simulink model "controlPC2"  (R2015b)
settings: Solver=ode45  StartTime=0.0  StopTime=100  RelTol=1e-3
values from neighbouring files (symbols this model uses):
  Kf = 20    [parametros.m]    (also in ploteo.m)
  Kpi = 0.014    [parametros.m]    (also in ploteo.m)
  T = 0.04    [parametros.m]    (also in ploteo.m)
  Ti = 0.25    [parametros.m]    (also in ploteo.m)
settings Model: Creator=Sony  LastModifiedBy=n421
settings DataIOCC: SaveFormat=Array
settings OptimizationCC: ExpressionDepthLimit=2147483647
settings DebuggingCC: UnderspecifiedInitializationDetection=Classic  MergeDetectMultiDrivingBlocksExec=none  SolverPrmCheckMsg=warning  StateNameClashWarn=warning
settings HardwareCC: ProdBitPerPointer=32  ProdLargestAtomicFloat=None  ProdIntDivRoundTo=Undefined  ProdEndianess=Unspecified  ProdWordSize=32  ProdHWDeviceType=32-bit Generic
settings GRTTargetCC: GeneratePreprocessorConditionals=Disable all
settings ConfigComp: CovModelRefEnable=Off

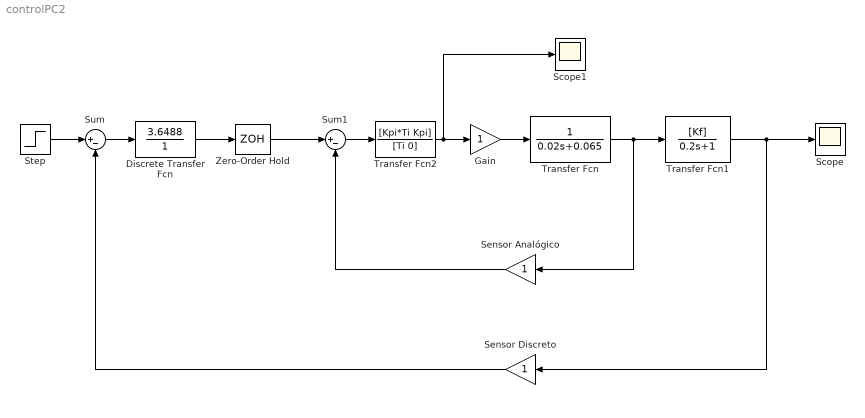
== system controlPC2 ==
  Discrete Transfer Fcn : DiscreteTransferFcn  Numerator=[3.6488]  Denominator=[1]  SampleTime=T
  Gain : Gain
  Scope : Scope
  Scope1 : Scope
  Sensor Analógico : Gain
  Sensor Discreto : Gain
  Step : Step  SampleTime=0
  Sum : Sum  Inputs=|+-
  Sum1 : Sum  Inputs=|+-
  Transfer Fcn : TransferFcn  Denominator=[0.02 0.065]
  Transfer Fcn1 : TransferFcn  Numerator=[Kf]  Denominator=[0.2 1]
  Transfer Fcn2 : TransferFcn  Numerator=[Kpi*Ti Kpi]  Denominator=[Ti 0]
  Zero-Order Hold : ZeroOrderHold  SampleTime=T
  wires:
  Transfer Fcn/1 -> Sensor Analógico/1, Transfer Fcn1/1
  Gain/1 -> Transfer Fcn/1
  Transfer Fcn1/1 -> Sensor Discreto/1, Scope/1
  Step/1 -> Sum/1
  Sensor Discreto/1 -> Sum/2
  Sum1/1 -> Transfer Fcn2/1
  Sensor Analógico/1 -> Sum1/2
  Transfer Fcn2/1 -> Scope1/1, Gain/1
  Zero-Order Hold/1 -> Sum1/1
  Sum/1 -> Discrete Transfer Fcn/1
  Discrete Transfer Fcn/1 -> Zero-Order Hold/1
